simulink library "hmi_menu_core_01_model"  (Simulink 7.0)
settings Model: Creator=jpradeep  LastModifiedBy=arajase2

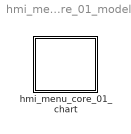
== system hmi_menu_core_01_model ==
  hmi_menu_core_01_chart : Stateflow chart

== stateflow chart hmi_menu_core_01_chart ==
  settings: executeAtInitialization=1  initializeOutput=1
  state hmi_menu_chart_Menu_FSTimeout [function]
    (junction 113) -> (junction 37)
    (junction 110) -> (junction 111) [order 1] : [!(in(HMI_MENU_WAIT_ST))]
        | {HMI_MENU_FS_REPEAT_TIMEOUT_EV;}
    (default) -> (junction 110)
    (junction 110) -> (junction 112) [order 2] : {HMI_MENU_FS_REPEAT_TIMER_EV;}
    (junction 112) -> (junction 113)
    (junction 111) -> (junction 113)
  state return_value = hmi_menu_chart_FS_btn_result [function]
    (default) -> (junction 70) : {
        |  return_value = l_get_btn_result_U8;
        | }
  state ret_status_BOOL = hmi_menu_chart_is_FS_st [function]
    (default) -> (junction 39) : {ret_status_BOOL = ((in(HMI_MENU_SCROLL_ST)));}
  state hmi_menu_chart_anim_started [function]
    (default) -> (junction 54) : {send(HMI_MENU_ANIM_STARTED_EV,HMI_MENU_ANIM_ST);}
  state hmi_menu_chart_close [function]
    (default) -> (junction 53) : {HMI_MENU_CLOSE_EV;}
  state hmi_menu_chart_Menu_open(p_menu_id_U8,p_cb_return_val_U16) [function]
    (default) -> (junction 47)
    (junction 47) -> (junction 58) [order 1] : [in(HMI_MENU_INACTIVE_ST)]
        | {l_menu_action_output_U16 = p_cb_return_val_U16;
        |  l_menu_id_U8 = p_menu_id_U8;
        |  HMI_MENU_OPEN_EV;}
    (junction 47) -> (junction 59) [order 2] : {l_menu_id_U8 = p_menu_id_U8;}
    (junction 58) -> (junction 60)
    (junction 60) -> (junction 59)
  state hmi_menu_chart_FS_Btn_process(p_menu_ID_U8, p_button_cmd_U16) [function]
    (junction 71) -> (junction 69)
    (junction 65) -> (junction 68) [order 1] : [hmi_menu_logic_FS_check_is_Btn_rel(p_button_cmd_U16) == TRUE]
        | {l_btn_cmd_U16  = p_button_cmd_U16;
        |  l_menu_id_U8 = p_menu_ID_U8;
        | HMI_MENU_FS_BTN_REL_EV;}
    (junction 65) -> (junction 69) [order 2]
    (junction 122) -> (junction 65) : {
        |     $#ifdef HMI_MENU_FAST_SCROLL_ENABLE$
        | }
    (junction 69) -> (junction 74) : {
        | $#endif$
        | }
    (junction 68) -> (junction 71)
    (junction 73) -> (junction 122) [order 2]
    (default) -> (junction 73)
    (junction 73) -> (junction 72) [order 1] : [in(HMI_MENU_FAST_SCROLL_INACTIVE_ST)]
        | {l_btn_cmd_U16  = p_button_cmd_U16;
        |  l_menu_id_U8 = p_menu_ID_U8;
        |  HMI_MENU_FS_BTN_EV;}
  state hmi_menu_chart_DataAvailable [function]
    (default) -> (junction 44) : {HMI_MENU_DATA_AVAIL_EV;}
  state hmi_menu_chart_anim_exit [function]
    (default) -> (junction 77) : {send(HMI_MENU_ANIM_EXIT_EV, HMI_MENU_ANIM_ST);}
  state hmi_menu_chart_Wait_temp_timeout [function]
    (default) -> (junction 62) : {HMI_MENU_WAIT_TEMP_TIMEOUT_EV;}
  state HMI_MENU_LOGIC_ST [parallel]
    entry:
    l_menu_action_output_U16   = 0;
    l_menu_action_U8                 = 0;
    $#ifdef HMI_MENU_FAST_SCROLL_ENABLE$
    l_repeat_count = 0;
    l_start_timer_value_U8 = 0;
    l_btn_cmd_U16 = 0;
    l_btn_rel_in_fast_scroll = 0;
    l_btn_status_BOOL = 0;
    $#endif$
    settings: executionOrder=1
    state HMI_MENU_INACTIVE_ST
    state HMI_MENU_ACTIVE_ST
      entry:
      fast_scroll_active = FALSE;
      fast_scroll_active_rel = FALSE;
    state HMI_MENU_SCROLL_ST
      entry:
      hmi_menu_fast_scroll_trigger();
      state hmi_menu_fast_scroll_trigger [function]
        (junction 125) -> (junction 45)
        (default) -> (junction 124)
        (junction 124) -> (junction 125) [order 1] : [fast_scroll_active == FALSE]
            | {
            |   hmi_menu_logic_activate_animation( l_menu_id_U8, l_menu_action_output_U16);
            |   fast_scroll_active = TRUE;
            | }
        (junction 124) -> (junction 35) [order 2]
        (junction 35) -> (junction 45) [order 1] : [fast_scroll_active_rel == TRUE]
            | {fast_scroll_active = FALSE;
            |  fast_scroll_active_rel = FALSE}
        (junction 45) -> (junction 41)
        (junction 46) -> (junction 41)
        (junction 35) -> (junction 46) [order 2] : /* Do Nothing*/
            | /* QAC 8.1.2 Fix*/
        (junction 41) -> (junction 121)
    state HMI_MENU_WAIT_ST
      exit:
      hmi_menu_logic_stop_timer(MENU_CORE_WAIT_TIMER,l_menu_id_U8);
      state HMI_MENU_WAIT_TEMP_TMR_ST
        entry:
        hmi_menu_logic_start_timer(MENU_CORE_WAIT_TIMER,l_menu_id_U8);
      state HMI_MENU_WAIT_ACTIVE_ST
        state HMI_MENU_WAIT_FOR_ANIM_EXIT
        state HMI_MENU_WAIT_ANIM_RUNNING_ST
          entry:
          hmi_menu_logic_stop_timer(MENU_CORE_WAIT_TIMER,l_menu_id_U8);
          hmi_menu_logic_activate_animation(l_menu_id_U8,MENU_CB_ACTION_WAIT);
          exit:
          hmi_menu_logic_deactivate_animation(l_menu_id_U8,MENU_CB_ACTION_WAIT);
          fast_scroll_active_rel = TRUE;
        HMI_MENU_WAIT_FOR_ANIM_EXIT -> HMI_MENU_WAIT_ANIM_RUNNING_ST : HMI_MENU_WAIT_ANIM_EXIT_EV
        (default) -> (junction 75)
        (junction 83) -> HMI_MENU_WAIT_ANIM_RUNNING_ST
        (junction 75) -> (junction 83) [order 1] : [in(HMI_MENU_ANIM_INACTIVE_ST)]
        (junction 75) -> HMI_MENU_WAIT_FOR_ANIM_EXIT [order 2]
      (default) -> HMI_MENU_WAIT_TEMP_TMR_ST
      HMI_MENU_WAIT_TEMP_TMR_ST -> HMI_MENU_WAIT_ACTIVE_ST : HMI_MENU_WAIT_TEMP_TIMEOUT_EV
    (junction 88) -> HMI_MENU_ACTIVE_ST [order 2]
    (junction 64) -> (junction 89) : {l_menu_action_output_U16 = hmi_menu_logic_process_menu_action(l_menu_id_U8, l_menu_action_U8);}
    (junction 84) -> (junction 85) : /*for MENU_CB_ACTION_ANIMATION|MENU_CB_ACTION_COMPLETED*/
    (junction 88) -> (junction 123) [order 1] : [hmi_menu_logic_MenuIsOpen(l_menu_id_U8) == FALSE]
    (junction 63) -> (junction 61) [order 2] : [hmi_menu_logic_is_menu_action_allowed_in_anim_state(l_menu_action_U8) == TRUE]
    (junction 85) -> (junction 96)
    (junction 61) -> (junction 66)
    (junction 66) -> (junction 64)
    (default) -> HMI_MENU_INACTIVE_ST
    (junction 63) -> (junction 64) [order 1] : [in(HMI_MENU_ANIM_INACTIVE_ST)]
    HMI_MENU_LOGIC_ST -> HMI_MENU_INACTIVE_ST [order 1] : HMI_MENU_CLOSE_EV
    HMI_MENU_INACTIVE_ST -> (junction 86) : HMI_MENU_OPEN_EV
    (junction 86) -> (junction 87) [order 1] : [l_menu_action_output_U16 == MENU_CB_ACTION_COMPLETED]
    (junction 87) -> HMI_MENU_ACTIVE_ST
    (junction 86) -> (junction 91) [order 2]
    (junction 123) -> HMI_MENU_INACTIVE_ST
    (junction 94) -> (junction 88)
    HMI_MENU_ACTIVE_ST -> (junction 63) : HMI_MENU_BTN_ACTIONS_EV
    (junction 90) -> (junction 89)
    (junction 92) -> (junction 90)
    (junction 89) -> (junction 93)
    HMI_MENU_SCROLL_ST -> (junction 92) [order 1] : HMI_MENU_BTN_ACTIONS_EV
        | {l_menu_action_output_U16 = hmi_menu_logic_process_menu_action(l_menu_id_U8, l_menu_action_U8);}
    (junction 91) -> (junction 93)
    (junction 93) -> HMI_MENU_SCROLL_ST [order 1] : [l_menu_action_output_U16 ==  MENU_CB_ACTION_FASTUP || ...
        |  l_menu_action_output_U16 ==  MENU_CB_ACTION_FASTDOWN]
    (junction 93) -> (junction 99) [order 2]
    (junction 95) -> (junction 92)
    (junction 96) -> (junction 94)
    HMI_MENU_SCROLL_ST -> (junction 95) [order 2] : HMI_MENU_BTN_MC_RELEASE_EV
        | {
        | $#ifdef HMI_MENU_FAST_SCROLL_ENABLE$
        | l_menu_action_output_U16 = hmi_menu_logic_MenuCompletion(l_menu_id_U8);
        | $#else$
        | l_menu_action_output_U16 = hmi_menu_logic_MenuCompletion();
        | $#endif$
        | /* hmi_menu_chart_FS_end_action();*/
        |  fast_scroll_active = FALSE;}
    (junction 98) -> (junction 95) : {l_menu_action_output_U16 = hmi_menu_logic_MenuDataAvailable(l_menu_id_U8);}
    HMI_MENU_WAIT_ST -> (junction 97) : HMI_MENU_DATA_AVAIL_EV
    (junction 97) -> (junction 98) [order 2]
    (junction 99) -> HMI_MENU_WAIT_ST [order 1] : [l_menu_action_output_U16 ==  MENU_CB_ACTION_WAIT]
    (junction 97) -> (junction 100) [order 1] : [l_btn_rel_in_fast_scroll != FALSE]
        | {l_btn_rel_in_fast_scroll = FALSE;
        | $#ifdef HMI_MENU_FAST_SCROLL_ENABLE$
        |    hmi_menu_logic_Set_MenuState(l_menu_id_U8,MENU_STATE_NORMAL);
        |    fl_cb_result     = hmi_menu_logic_MenuCompletion(l_menu_id_U8);
        | $#else$
        |    fl_cb_result     = hmi_menu_logic_MenuCompletion();
        | $#endif$}
    (junction 101) -> (junction 98)
    (junction 99) -> (junction 84) [order 2]
    (junction 100) -> (junction 101) [order 2]
    (junction 100) -> HMI_MENU_WAIT_ST [order 1] : [fl_cb_result == MENU_CB_ACTION_WAIT]
        | {hmi_menu_logic_deactivate_animation(l_menu_id_U8,MENU_CB_ACTION_FASTUP);}
    HMI_MENU_LOGIC_ST -> (junction 91) [order 2] : HMI_MENU_REBUILD_EV
  state HMI_MENU_ANIM_ST [parallel]
    settings: executionOrder=2
    state HMI_MENU_ANIM_INACTIVE_ST
      entry:
      send(HMI_MENU_WAIT_ANIM_EXIT_EV, HMI_MENU_WAIT_FOR_ANIM_EXIT);
    state HMI_MENU_ANIM_ACTIVE_ST
    HMI_MENU_ANIM_ACTIVE_ST -> HMI_MENU_ANIM_INACTIVE_ST : HMI_MENU_ANIM_EXIT_EV
    HMI_MENU_ANIM_INACTIVE_ST -> HMI_MENU_ANIM_ACTIVE_ST : /* animation started by view manager and vm is in anim state*/
        | HMI_MENU_ANIM_STARTED_EV
    HMI_MENU_ANIM_ST -> HMI_MENU_ANIM_INACTIVE_ST : HMI_MENU_CLOSE_EV
    (default) -> HMI_MENU_ANIM_INACTIVE_ST
  state hmi_menu_fast_scroll_inactive [function]
    (junction 114) -> (junction 116) [order 2]
    (junction 114) -> (junction 117) [order 1] : [in(HMI_MENU_FAST_SCROLL_ACTIVE_ST)]
        | {HMI_MENU_FS_INACTIVE_EV;}
    (default) -> (junction 114)
    (junction 117) -> (junction 118) [order 1] : [fast_scroll_active == TRUE]
    (junction 117) -> (junction 119) [order 2]
    (junction 118) -> (junction 120) : {hmi_menu_logic_deactivate_animation(l_menu_id_U8,MENU_CB_ACTION_FASTUP);
        |   fast_scroll_active = FALSE;}
    (junction 119) -> (junction 120)
    (junction 120) -> (junction 115)
    (junction 115) -> (junction 116)
  state hmi_menu_chart_menu_rebuild(fl_menu_cb_output_U16) [function]
    (junction 76) -> (junction 56) [order 2]
    (default) -> (junction 76)
    (junction 76) -> (junction 81) [order 1] : [!in(HMI_MENU_INACTIVE_ST)]
        | {l_menu_action_output_U16 = fl_menu_cb_output_U16;
        |  HMI_MENU_REBUILD_EV;}
  state HMI_MENU_FAST_SCROLL_ST [parallel]
    settings: executionOrder=3
    state HMI_MENU_FAST_SCROLL_INACTIVE_ST
    state HMI_MENU_FAST_SCROLL_LIST_END_ST
      entry:
      hmi_menu_logic_stop_timer(MENU_CORE_FASTSCROLL_RUN_WAIT_TIMER,l_menu_id_U8);
      hmi_menu_logic_deactivate_animation(l_menu_id_U8, l_menu_action_output_U16);
      l_repeat_count = 0;
      l_menu_state = MENU_STATE_NORMAL;
      hmi_menu_logic_Set_MenuState(l_menu_id_U8,MENU_STATE_NORMAL);
    state HMI_MENU_FAST_SCROLL_ACTIVE_ST
      entry:
      $#ifdef HMI_MENU_FAST_SCROLL_ENABLE$
      l_get_btn_result_U8 = hmi_menu_button_handler(l_menu_id_U8, l_btn_cmd_U16, l_menu_state);
      $#else$
      l_get_btn_result_U8 = MENU_CB_ACTION_COMPLETED;
      $#endif$
      on HMI_MENU_FS_REPEAT_TIMER_EV:
      hmi_menu_logic_start_timer(MENU_CORE_FASTSCROLL_RUN_WAIT_TIMER,l_menu_id_U8);
      exit:
      /*hmi_menu_logic_stop_timer(MENU_CORE_FASTSCROLL_RUN_WAIT_TIMER,l_menu_id_U8);*/
    HMI_MENU_FAST_SCROLL_ST -> HMI_MENU_FAST_SCROLL_INACTIVE_ST : HMI_MENU_CLOSE_EV
    HMI_MENU_FAST_SCROLL_LIST_END_ST -> HMI_MENU_FAST_SCROLL_INACTIVE_ST : HMI_MENU_FS_BTN_REL_EV
    (junction 38) -> (junction 67) [order 1] : [l_menu_state == MENU_STATE_FAST]
        | {
        |  hmi_menu_logic_deactivate_animation(l_menu_id_U8, l_menu_action_output_U16);
        |  l_menu_state = MENU_STATE_NORMAL;
        |  hmi_menu_logic_Set_MenuState(l_menu_id_U8,MENU_STATE_NORMAL);
        | }
    (junction 38) -> HMI_MENU_FAST_SCROLL_INACTIVE_ST [order 2] : {l_menu_state = MENU_STATE_NORMAL;
        | hmi_menu_logic_Set_MenuState(l_menu_id_U8,MENU_STATE_NORMAL);}
    (junction 67) -> HMI_MENU_FAST_SCROLL_INACTIVE_ST
    (junction 103) -> (junction 102)
    (junction 105) -> (junction 104)
    (junction 106) -> (junction 105) [order 2]
    (junction 107) -> (junction 103) [order 2] : {
        |   l_menu_state = MENU_STATE_NORMAL;
        |   hmi_menu_logic_start_timer(MENU_CORE_FASTSCROLL_CNT_INCR_TIMER,l_menu_id_U8);
        |   l_repeat_count++;
        |   l_btn_status_BOOL = HMI_MENU_BTN_STATUS_IN;
        | }
    (junction 104) -> (junction 108)
    (junction 107) -> (junction 106) [order 1] : [(l_repeat_count > HMI_MENU_SCROLL_REPEAT_COUNT) &&...
        |  (hmi_menu_logic_is_FS_Enabled(l_menu_id_U8) == TRUE)]
        | {
        |   l_menu_state = MENU_STATE_FAST;
        |   hmi_menu_logic_start_timer(MENU_CORE_FASTSCROLL_RUN_WAIT_TIMER,l_menu_id_U8);
        | }
    (junction 106) -> (junction 108) [order 1] : [ l_btn_status_BOOL == HMI_MENU_BTN_STATUS_IN]
        |  {
        |     l_btn_status_BOOL = HMI_MENU_BTN_STATUS_LONG;
        | $#ifdef HMI_MENU_FAST_SCROLL_ENABLE$
        |     l_btn_cmd_U16 = hmi_menu_logic_FS_convert_Btn_status(l_btn_status_BOOL, l_btn_cmd_U16);
        | $#else$
        |     l_btn_cmd_U16 = MENU_BTN_INVALID;
        | $#endif$
        |  }
    HMI_MENU_FAST_SCROLL_ACTIVE_ST -> (junction 107) [order 1] : HMI_MENU_FS_REPEAT_TIMEOUT_EV
        | {hmi_menu_logic_stop_timer(MENU_CORE_FASTSCROLL_RUN_WAIT_TIMER,l_menu_id_U8);}
    (junction 108) -> (junction 109)
    (junction 109) -> HMI_MENU_FAST_SCROLL_ACTIVE_ST
    HMI_MENU_FAST_SCROLL_INACTIVE_ST -> HMI_MENU_FAST_SCROLL_ACTIVE_ST : HMI_MENU_FS_BTN_EV
        | {
        |    l_repeat_count = 1;
        |    l_menu_state = MENU_STATE_NORMAL;
        |    hmi_menu_logic_start_timer(MENU_CORE_FASTSCROLL_CNT_START_TIMER,l_menu_id_U8);
        | }
    HMI_MENU_FAST_SCROLL_ACTIVE_ST -> (junction 38) [order 3] : HMI_MENU_FS_BTN_REL_EV
        | {
        |   hmi_menu_logic_stop_timer(MENU_CORE_FASTSCROLL_RUN_WAIT_TIMER,l_menu_id_U8);
        | $#ifdef HMI_MENU_FAST_SCROLL_ENABLE$
        | l_get_btn_result_U8 = hmi_menu_button_handler(l_menu_id_U8, l_btn_cmd_U16, l_menu_state);
        | $#else$
        | l_get_btn_result_U8 = MENU_CB_ACTION_COMPLETED;
        | $#endif$
        |  l_repeat_count = 0;
        | }
    HMI_MENU_FAST_SCROLL_ACTIVE_ST -> HMI_MENU_FAST_SCROLL_LIST_END_ST [order 2] : HMI_MENU_FS_INACTIVE_EV
    (default) -> HMI_MENU_FAST_SCROLL_INACTIVE_ST
    (junction 102) -> (junction 104)
  state ret_status_BOOL = hmi_menu_chart_is_anim_st [function]
    (default) -> (junction 57) : {ret_status_BOOL = (in(HMI_MENU_ANIM_ACTIVE_ST));}
  state return_btn_result_U8 = hmi_menu_chart_Btn_trigger(p_menu_ID_U8, p_menu_btn_action_U8, p_menu_state) [function]
    state return_st = hmi_menu_chart_check_MC_rel [function]
      (junction 48) -> (junction 51)
      (junction 50) -> (junction 49) [order 1] : [(l_menu_action_U8 == MENU_ACTION_UP_RELEASE) ||...
          |  (l_menu_action_U8 == MENU_ACTION_DOWN_RELEASE) ||...
          |  (l_menu_action_U8 ==MENU_ACTION_LEFT_RELEASE)||...
          |  (l_menu_action_U8 == MENU_ACTION_RIGHT_RELEASE)]
      (junction 50) -> (junction 51) [order 2] : {return_st = FALSE;}
      (junction 49) -> (junction 48) : {return_st = TRUE;}
      (default) -> (junction 50)
    (default) -> (junction 55)
    (junction 78) -> (junction 42) : {
        |   return_btn_result_U8 = MENU_BTN_ABSORBED;
        | }
    (junction 80) -> (junction 78)
    (junction 55) -> (junction 43) [order 2] : {return_btn_result_U8 = MENU_BTN_NONE;}
    (junction 79) -> (junction 52) : {l_btn_rel_in_fast_scroll = TRUE;}
    (junction 52) -> (junction 80)
    (junction 40) -> (junction 36)
    (junction 55) -> (junction 40) [order 1] : [ in(HMI_MENU_ACTIVE_ST) || in(HMI_MENU_SCROLL_ST) || in(HMI_MENU_WAIT_ST)]
        | { l_menu_action_U8 = p_menu_btn_action_U8;
        |   l_menu_id_U8 = p_menu_ID_U8;}
    (junction 82) -> (junction 80) [order 2] : {HMI_MENU_BTN_MC_RELEASE_EV;}
    (junction 36) -> (junction 78) [order 2] : {HMI_MENU_BTN_ACTIONS_EV;}
    (junction 82) -> (junction 79) [order 1] : [(in(HMI_MENU_WAIT_ST)) &&...
        |  (p_menu_state == MENU_STATE_FAST)]
    (junction 36) -> (junction 82) [order 1] : [(in(HMI_MENU_SCROLL_ST) || in(HMI_MENU_WAIT_ST)) &&...
        |  (TRUE == hmi_menu_chart_check_MC_rel())]
    (junction 42) -> (junction 43)
  data: fl_get_Menu_Timer_val_U8 local uint8; return_value function_output uint8; ret_status_BOOL function_output boolean; result local boolean; p_menu_id_U8 function_input uint8; p_cb_return_val_U16 function_input uint16; return_st function_output boolean; p_menu_ID_U8 function_input uint8; p_button_cmd_U16 function_input uint16; fl_cb_result local uint16; fl_menu_cb_output_U16 function_input uint16; ret_status_BOOL function_output boolean; p_menu_ID_U8 function_input uint8; p_menu_btn_action_U8 function_input uint8; return_btn_result_U8 function_output uint8; p_menu_state function_input uint8; l_menu_action_U8 local uint8; l_menu_action_output_U16 local uint16; l_get_btn_result_U8 local uint8; l_btn_cmd_U16 local uint16; l_menu_id_U8 local uint8; l_btn_rel_in_fast_scroll local boolean; l_start_timer_value_U8 local uint16; l_menu_state local uint8; l_repeat_count local uint8; l_btn_status_BOOL local boolean; fl_get_FS_exit_status_BOOL local boolean; fast_scroll_active local boolean; fast_scroll_active_rel local boolean; temp_wait_flag local boolean
  events: HMI_MENU_OPEN_EV local EITHER_EDGE_EVENT; HMI_MENU_CLOSE_EV local EITHER_EDGE_EVENT; HMI_MENU_DATA_AVAIL_EV local EITHER_EDGE_EVENT; HMI_MENU_ANIM_EXIT_EV local EITHER_EDGE_EVENT; HMI_MENU_BTN_ACTIONS_EV local EITHER_EDGE_EVENT; HMI_MENU_BTN_MC_RELEASE_EV local EITHER_EDGE_EVENT; HMI_MENU_FS_BTN_EV local EITHER_EDGE_EVENT; HMI_MENU_FS_BTN_REL_EV local EITHER_EDGE_EVENT; HMI_MENU_FS_REPEAT_TIMEOUT_EV local EITHER_EDGE_EVENT; HMI_MENU_OPEN_INSTANCE_EV local EITHER_EDGE_EVENT; HMI_MENU_WAIT_TEMP_TIMEOUT_EV local EITHER_EDGE_EVENT; HMI_MENU_FS_REPEAT_TIMER_EV local EITHER_EDGE_EVENT; HMI_MENU_FS_INACTIVE_EV local EITHER_EDGE_EVENT; HMI_MENU_REBUILD_EV local EITHER_EDGE_EVENT; HMI_MENU_ANIM_STARTED_EV local EITHER_EDGE_EVENT; HMI_MENU_WAIT_ANIM_EXIT_EV local EITHER_EDGE_EVENT
